simulink model "single_battery_reDCDC"  (R2023b)
settings: Solver=VariableStepAuto  StartTime=0.0  StopTime=0.2  RelTol=1e-3
undefined symbols (not defined in the file): Ion, Lithium
libraries: spsSeriesRLCBranchLib x3, spsMosfetLib x2, spsOnDelayLib x2, spsVoltageMeasurementLib x2, spsBatteryLib x1, spsCurrentMeasurementLib x1, slpidlib x1, spsTriangleGeneratorLib x1, spspowerguiLib x1
settings Model: Creator=zhaoxu  LastModifiedBy=zhaoxu

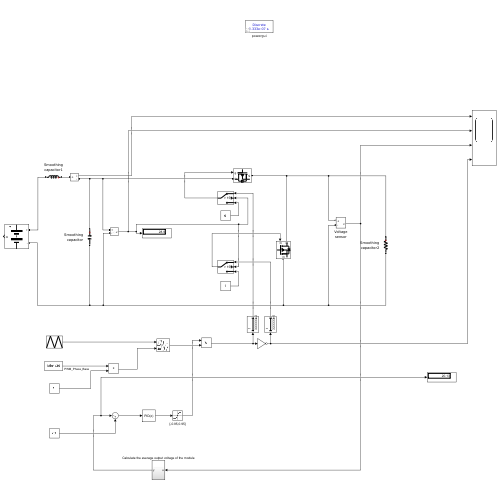
[thumbnail: Simulink's stored preview of the top-level diagram]
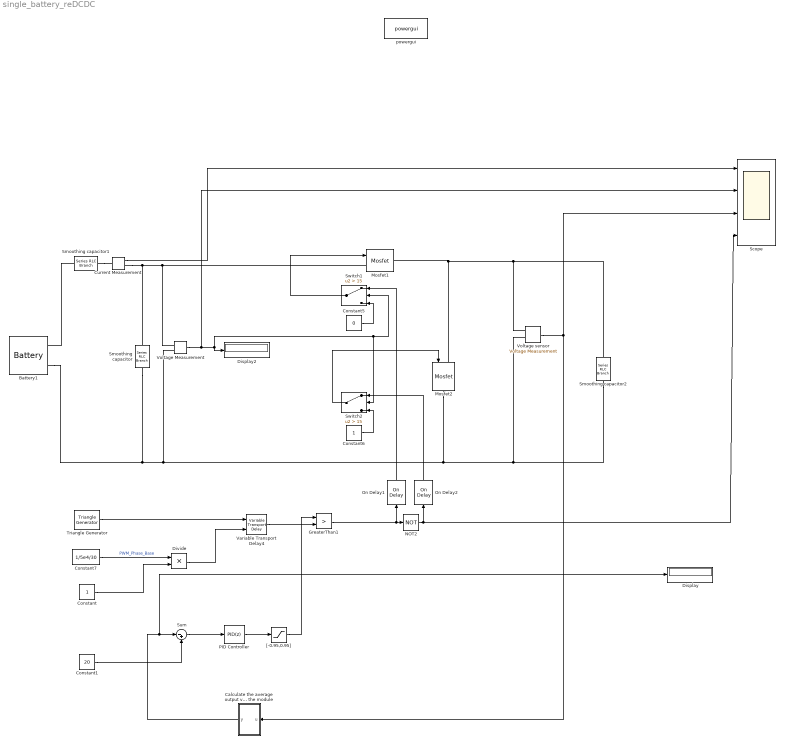
== system single_battery_reDCDC ==
  Battery1 : spsBatteryLib/Battery  BatType=Lithium-Ion  ShowTempParam=off  ThermalPreset=no  ShowAgeParam=off  NomV=25.6  NomQ=50  SOC=70  Batt_Tr=30  PresetModel=on  MaxQ=50  MinV=19.2  FullV=29.7981  Dis_rate=21.7391  R=0.00512  Normal_OP=45.2174  expZone="[27.6579      2.45652]"  current=[6.5 13 32.5]  Units=Ampere-hour  Tci=20  NomT=20  T2=-30  MaxQ2=4.8  FullV2=7.1  Normal_OP2=5.655  expZone2="[6.58           1]"  Rca=0.6  ti=2000  Dp=0  Neq0=0  Tsim=1e6  Ta1=25  Qeol=5.4*0.9  Reol=0.013333*1.2  Char_age=[2.3478, 3]  Dis_age=[2.3478, 10]  N1=1500  N2=10500  N3=1000  N4=1400  Ta2=45  N5=950
  Calculate the average output voltage of the module : Subsystem
  Constant : Constant
  Constant1 : Constant  Value=20
  Constant5 : Constant  Value=0
  Constant6 : Constant
  Constant7 : Constant  Value=1/5e4/30
  Current Measurement : spsCurrentMeasurementLib/Current Measurement  PhasorSimulation=off  OutputType=Complex  PSBequivalent=0
  Display : Display
  Display2 : Display
  Divide : Product  Inputs=**
  GreaterThan1 : RelationalOperator  Operator=>  OutDataTypeStr=boolean  RndMeth=Simplest  InputSameDT=off
  Mosfet1 : spsMosfetLib/Mosfet  Ron=1.7e-3  Lon=0  Rd=0.01  Vfd=0.9  IC=0  Rs=1e5  Cs=inf  Measurements=off
  Mosfet2 : spsMosfetLib/Mosfet  Ron=1.7e-3  Lon=0  Rd=0.01  Vfd=0.9  IC=0  Rs=1e5  Cs=inf  Measurements=off
  NOT2 : Logic  Operator=NOT  IconShape=distinctive  AllPortsSameDT=off  OutDataTypeStr=boolean
  On Delay1 : spsOnDelayLib/On Delay  DelayType=On delay  delay=1/5e4/60  ic=0  Ts=0
  On Delay2 : spsOnDelayLib/On Delay  DelayType=On delay  delay=1/5e4/60  ic=0  Ts=0
  PID Controller : slpidlib/PID Controller  Controller=PID  Form=Parallel  TimeDomain=Discrete-time  UseExternalTs=off  SampleTime=1e-4  IntegratorMethod=Forward Euler  FilterMethod=Forward Euler  ControllerParametersSource=internal  P=0.05  I=9  UseKiTs=off  D=0.0001  N=100  UseFilter=on  TunerSelectOption=Transfer Function Based (PID Tuner App)  InitialConditionSource=internal  InitialConditionForIntegrator=0  InitialConditionForFilter=0  DifferentiatorICPrevScaledInput=0  ExternalReset=none  TrackingMode=off  Kt=1  LimitOutput=off  SatLimitsSource=internal  UpperSaturationLimit=inf  LowerSaturationLimit=-inf  LinearizeAsGain=on  AntiWindupMode=none  Kb=1  LimitIntegrator=off  UpperIntegratorSaturationLimit=inf  LowerIntegratorSaturationLimit=-inf  POutMin=[]  POutMax=[]  IOutMin=[]  IOutMax=[]  DOutMin=[]  DOutMax=[]  NOutMin=[]  NOutMax=[]  SumOutMin=[]  SumOutMax=[]  SaturationOutMin=[]  SaturationOutMax=[]  PParamMin=[]  PParamMax=[]  IParamMin=[]  IParamMax=[]  DParamMin=[]  DParamMax=[]  NParamMin=[]  NParamMax=[]  KbParamMin=[]  KbParamMax=[]  KtParamMin=[]  KtParamMax=[]  KbOutMin=[]  KbOutMax=[]  KtOutMin=[]  KtOutMax=[]  IntegratorOutMin=[]  IntegratorOutMax=[]  FilterOutMin=[]  FilterOutMax=[]  SumI1OutMin=[]  SumI1OutMax=[]  SumI2OutMin=[]  SumI2OutMax=[]  SumI3OutMin=[]  SumI3OutMax=[]  SumI4OutMin=[]  SumI4OutMax=[]  SumDOutMin=[]  SumDOutMax=[]  DifferentiatorOutMin=[]  DifferentiatorOutMax=[]  FilterDiffOutCoefMin=[]  FilterDiffOutCoefMax=[]  ReciprocalOutMin=[]  ReciprocalOutMax=[]  SumDenOutMin=[]  SumDenOutMax=[]  SumNumOutMin=[]  SumNumOutMax=[]  DivideOutMin=[]  DivideOutMax=[]  UdiffTsProdOutMin=[]  UdiffTsProdOutMax=[]  NTsProdOutMin=[]  NTsProdOutMax=[]  UintegralTsProdOutMin=[]  UintegralTsProdOutMax=[]  UngainTsProdOutMin=[]  UngainTsProdOutMax=[]  ClampingZeroOutDataTypeStr=Inherit: Inherit via back propagation  ClampingZeroOutMin=[]  ClampingZeroOutMax=[]  FilterDenConstantOutDataTypeStr=Inherit: Inherit via back propagation  FilterDenConstantOutMin=[]  FilterDenConstantOutMax=[]  PCopyOutDataTypeStr=Inherit: Inherit via back propagation  PCopyOutMin=[]  PCopyOutMax=[]  NCopyOutDataTypeStr=Inherit: Inherit via back propagation  NCopyOutMin=[]  NCopyOutMax=[]  IntegratorContinuousStateAttributes=''  IntegratorStateMustResolveToSignalObject=off  IntegratorRTWStateStorageClass=Auto  FilterContinuousStateAttributes=''  FilterStateMustResolveToSignalObject=off  FilterRTWStateStorageClass=Auto  ParallelPVariant=InternalParameters  IdealPVariant=Disabled  IVariant=InternalParameters  DVariant=InternalParameters  IntegratorVariant=Discrete  SatVariant=Disabled  AWVariant=Passthrough  PCopyVariant=Disabled  TRVariant=Disabled  FdbkBlocksVariant=Forward  IdealPFdbkVariant=Disabled  SatFdbkVariant=Disabled  DerivativeFilterVariant=ForwardEulerFilter  NVariant=InternalParameters  NCopyVariant=Disabled  FilterICVariant=InternalICsFilter  IntegratorICVariant=InternalICs  ExternalResetVariant=Disabled  TRSumVariant=Passthrough  SumFdbkVariant=Disabled  SumVariant=Sum_PID  TsampFilterVariant=InternalTs  TsampNgainVariant=Passthrough  TsampIntegralVariant=Disabled_SignalSpec  ExternalSaturationOutDataTypeStr=Inherit: Same as second input
  Scope : Scope  NumInputPorts=4
  Smoothing capacitor : spsSeriesRLCBranchLib/Series RLC Branch  LConnTagsString=__new0  RConnTagsString=__new0  BranchType=C  Resistance=1  Inductance=1e-3  SetiL0=off  InitialCurrent=0  Capacitance=7.22e-5  Setx0=off  InitialVoltage=0  Measurements=None
  Smoothing capacitor1 : spsSeriesRLCBranchLib/Series RLC Branch  LConnTagsString=__new0  RConnTagsString=__new0  BranchType=L  Resistance=1  Inductance=2.5e-7  SetiL0=off  InitialCurrent=0  Capacitance=7.22e-5  Setx0=off  InitialVoltage=0  Measurements=None
  Smoothing capacitor2 : spsSeriesRLCBranchLib/Series RLC Branch  LConnTagsString=__new0  RConnTagsString=__new0  BranchType=R  Resistance=1  Inductance=1e-3  SetiL0=off  InitialCurrent=0  Capacitance=7.22e-5  Setx0=off  InitialVoltage=0  Measurements=None
  Sum : Sum  Inputs=|-+  InputSameDT=on  SaturateOnIntegerOverflow=on  OutDataTypeStr=Inherit: Same as first input
  Switch1 : Switch  Criteria=u2 > Threshold  Threshold=15  SaturateOnIntegerOverflow=off  InputSameDT=off
  Switch2 : Switch  Criteria=u2 > Threshold  Threshold=15  SaturateOnIntegerOverflow=off  InputSameDT=off
  Triangle Generator : spsTriangleGeneratorLib/Triangle Generator  Freq=50000  Phase=0  Ts=0
  Variable Transport Delay4 : VariableTransportDelay  MaximumDelay=10
  Voltage sensor : spsVoltageMeasurementLib/Voltage Measurement  PhasorSimulation=off  OutputType=Complex  PSBequivalent=0
  Voltage Measurement : spsVoltageMeasurementLib/Voltage Measurement  PhasorSimulation=off  OutputType=Complex  PSBequivalent=0
  "[-0.95,0.95]" : Saturate  UpperLimit=0.95  LowerLimit=-0.95
  powergui : spspowerguiLib/powergui  Priority=1  SimulationMode=Discrete  SampleTime=1/5e4/60  frequency=60  Iterations=50  frequencyindice=0  Pbase=100e6  ErrMax=1e-4  UnitsV=kV  UnitsW=MW  buscounter=0  FunctionMessages=off  echomessages=off  EnableUseOfTLC=off  CurrentSourceSwitches=off  DisableSnubberDevices=off  DisableRonSwitches=off  DisableVfSwitches=off  DisplayEquations=off  AutomaticDiscreteSolvers=off  SolverType=Tustin/Backward Euler (TBE)  Interpol=off  ExternalGateDelay=off  methode=off  Ts=100  x0status=blocks  SPID=on  SwTol=0  HookPort=off  NonlinearTolerance=1e-4  nMaxIteration=100  ContinueOnMaxIteration=off  RestoreLinks=warning  ResistiveCurrentMeasurement=off  Frange=[0:2:500]  Ylog=off  Xlog=on  ShowGrid=off  save=off  variable=ZData  structure=0  ZoomFFT=on  StartTime=0.0  cycles=1  DisplayStyle=1  fundamental=60  FreqAxis=off  MaxFrequency=1000  frequencyindicesteady=1  RmsSteady=1  display=off
  wires:
  Constant1/1 -> Sum/2
  On Delay2/1 -> Switch2/1
  GreaterThan1/1 -> On Delay1/1, NOT2/1
  Voltage sensor/1 -> Calculate the average output voltage of the module/1(u), Scope/3
  Variable Transport Delay4/1 -> GreaterThan1/2
  "[-0.95,0.95]"/1 -> GreaterThan1/1
  Constant5/1 -> Switch1/3
  Triangle Generator/1 -> Variable Transport Delay4/1
  On Delay1/1 -> Switch1/1
  Switch2/1 -> Mosfet2/1
  Divide/1 -> Variable Transport Delay4/2
  Voltage Measurement/1 -> Scope/2, Display2/1, Switch1/2, Switch2/2
  Switch1/1 -> Mosfet1/1
  PID Controller/1 -> "[-0.95,0.95]"/1
  Sum/1 -> PID Controller/1
  Constant6/1 -> Switch2/3
  Constant7/1 -> Divide/1  "PWM_Phase_Base"
  Constant/1 -> Divide/2
  Current Measurement/1 -> Scope/1
  NOT2/1 -> Scope/4, On Delay2/1
  Calculate the average output voltage of the module/1(y) -> Display/1, Sum/1
  connections:
  Voltage sensor/LConn2 -- Smoothing capacitor2/RConn1 -- Mosfet2/RConn1 -- Smoothing capacitor/RConn1 -- Battery1/LConn2 -- Voltage Measurement/LConn2
  Current Measurement/RConn1 -- Smoothing capacitor/LConn1 -- Mosfet1/LConn1 -- Voltage Measurement/LConn1
  Mosfet1/RConn1 -- Mosfet2/LConn1 -- Smoothing capacitor2/LConn1 -- Voltage sensor/LConn1
  Smoothing capacitor1/RConn1 -- Battery1/LConn1
  Smoothing capacitor1/LConn1 -- Current Measurement/LConn1

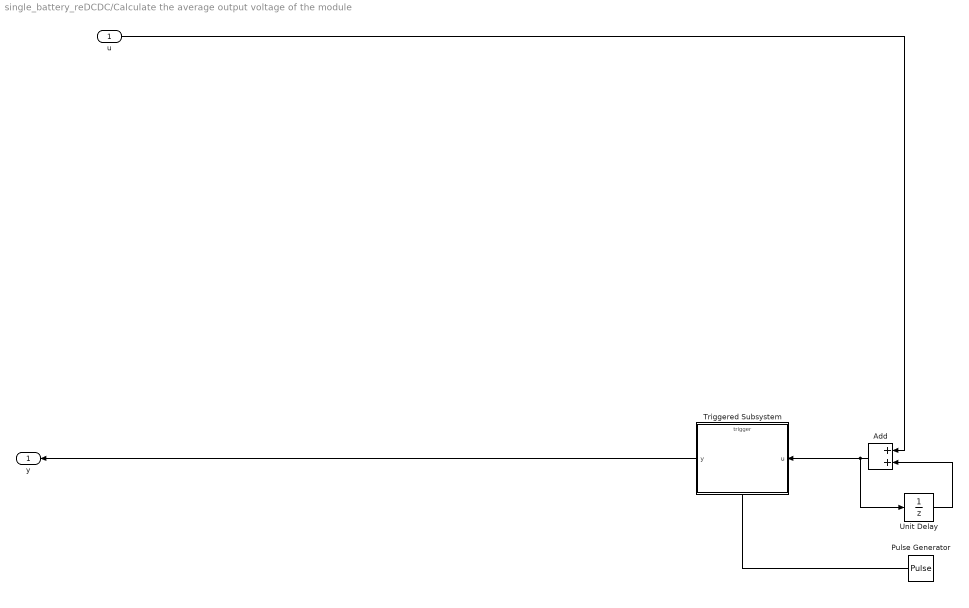
== system single_battery_reDCDC/Calculate the average output voltage of the module ==
  u : Inport
  Add : Sum
  Pulse Generator : DiscretePulseGenerator  PulseType=Time based  Period=1e-4  PulseWidth=50
  Triggered Subsystem : Subsystem  TreatAsAtomicUnit=on
  Unit Delay : UnitDelay  SampleTime=1/5e4/60  HasFrameUpgradeWarning=on
  y : Outport
  wires:
  Add/1 -> Unit Delay/1, Triggered Subsystem/1(u)
  Pulse Generator/1 -> Triggered Subsystem/Trigger
  Unit Delay/1 -> Add/2
  Triggered Subsystem/1(y) -> y/1
  u/1 -> Add/1

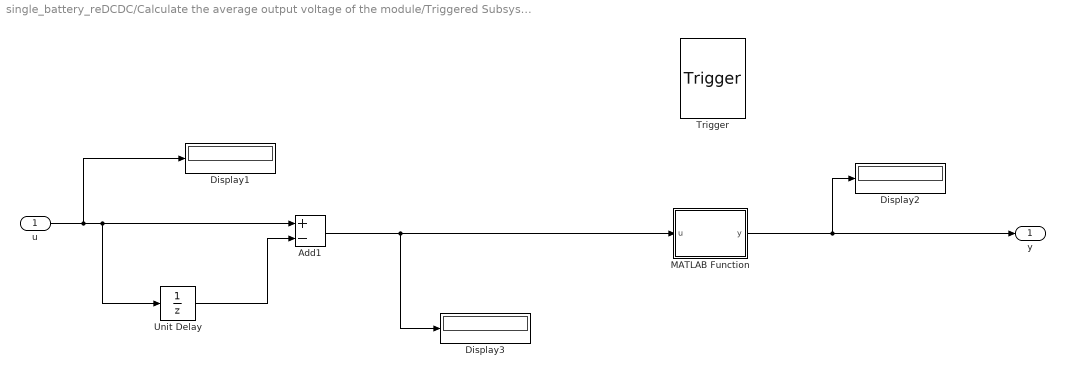
== system single_battery_reDCDC/Calculate the average output voltage of the module/Triggered Subsystem ==
  u : Inport
  Trigger : TriggerPort  VariantControl=(inherit)
  Add1 : Sum  Inputs=+-
  Display1 : Display
  Display2 : Display
  Display3 : Display
  MATLAB Function : MATLAB Function  TreatAsAtomicUnit=on
  Unit Delay : UnitDelay  SampleTime=-1  HasFrameUpgradeWarning=on
  y : Outport
  wires:
  MATLAB Function/1(y) -> Display2/1, y/1
  u/1 -> Display1/1, Unit Delay/1, Add1/1
  Add1/1 -> Display3/1, MATLAB Function/1(u)
  Unit Delay/1 -> Add1/2

== matlab function single_battery_reDCDC/Calculate the average output voltage of the module/Triggered Subsystem/MATLAB Function ==
  data: u input; y output
function y = fcn(u)
%#codegen

y = u / 300;
